simulink model "ATABEY_sistem_modeli"  (R2025b)
settings: Solver=VariableStepAuto  StartTime=0.0  StopTime=simTime  RelTol=1e-3
undefined symbols (not defined in the file or in its folder): uMotorMax, uMotorMin, uServoMax, uServoMin, x0
libraries: aerolibfltsims x1, aerolibanimutils x1
settings Model: Creator=erayacikgz  LastModifiedBy=erayacikgz

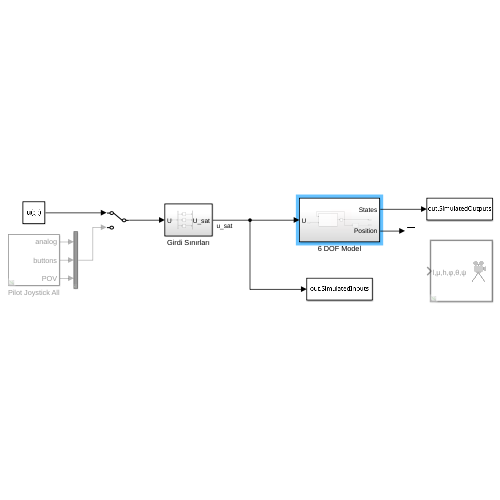
[thumbnail: Simulink's stored preview of the top-level diagram]
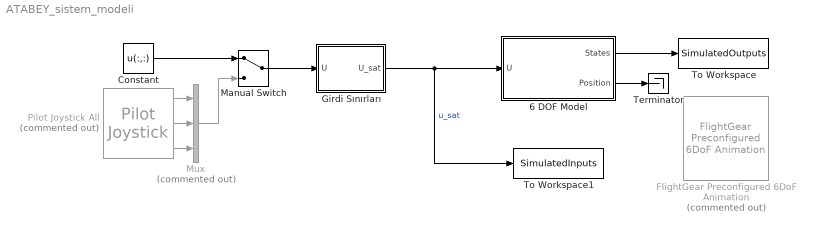
== system ATABEY_sistem_modeli ==
  6 DOF Model : Subsystem
  Constant : Constant  Value=u(:,:)
  FlightGear Preconfigured 6DoF Animation : aerolibfltsims/FlightGear Preconfigured 6DoF Animation  Commented=on  xFlightGearVersion=v2019.1  DestinationIpAddress=127.0.0.1  DestinationPort=5502  SampleTime=1/30  packetVersion=24
  Girdi Sınırları : Subsystem
  Manual Switch : ManualSwitch
  Mux : Mux  Commented=on  Inputs=3
  Pilot Joystick All : aerolibanimutils/Pilot Joystick  Commented=on  JoystickID=Joystick1  OutputConfiguration=AllOutputs  SampleTime=1/30
      settings: LibrarySourceBlock=aerolibanimutils/Pilot Joystick All
  Terminator : Terminator
  To Workspace : ToWorkspace  VariableName=SimulatedOutputs  SaveFormat=Timeseries  SampleTime=-1
  To Workspace1 : ToWorkspace  VariableName=SimulatedInputs  SaveFormat=Timeseries  SampleTime=-1
  wires:
  6 DOF Model/1(States) -> To Workspace/1
  Manual Switch/1 -> Girdi Sınırları/1(U)
  Constant/1 -> Manual Switch/1
  Pilot Joystick All/1 -> Mux/1
  Pilot Joystick All/2 -> Mux/2
  Pilot Joystick All/3 -> Mux/3
  Mux/1 -> Manual Switch/2
  6 DOF Model/2(Position) -> Terminator/1
  Girdi Sınırları/1(U_sat) -> To Workspace1/1, 6 DOF Model/1(U)  "u_sat"

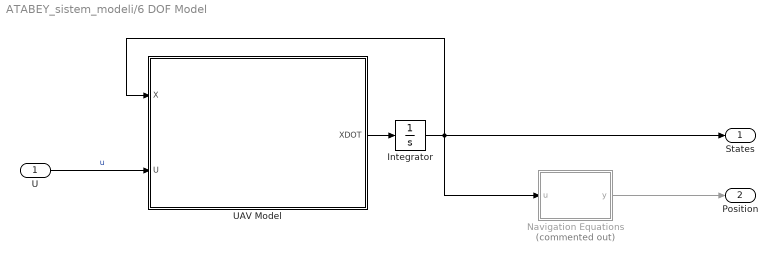
== system ATABEY_sistem_modeli/6 DOF Model ==
  U : Inport
  Integrator : Integrator  InitialCondition=x0(:,:)
  Navigation Equations : MATLAB Function  Commented=on  TreatAsAtomicUnit=on
  UAV Model : MATLAB Function  TreatAsAtomicUnit=on
  States : Outport
  Position : Outport  Port=2
  wires:
  U/1 -> UAV Model/2(U)  "u"
  Navigation Equations/1(y) -> Position/1
  UAV Model/1(XDOT) -> Integrator/1
  Integrator/1 -> States/1, Navigation Equations/1(u), UAV Model/1(X)

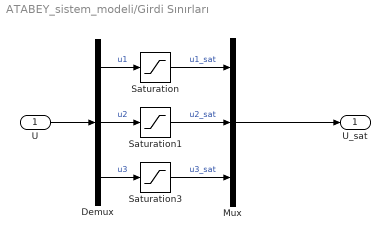
== system ATABEY_sistem_modeli/Girdi Sınırları ==
  U : Inport
  Demux : Demux  Outputs=3
  Mux : Mux  Inputs=3
  Saturation : Saturate  UpperLimit=uServoMax  LowerLimit=uServoMin
  Saturation1 : Saturate  UpperLimit=uServoMax  LowerLimit=uServoMin
  Saturation3 : Saturate  UpperLimit=uMotorMax  LowerLimit=uMotorMin
  U_sat : Outport
  wires:
  Mux/1 -> U_sat/1
  Demux/2 -> Saturation1/1  "u2"
  Saturation/1 -> Mux/1  "u1_sat"
  Saturation3/1 -> Mux/3  "u3_sat"
  U/1 -> Demux/1
  Demux/1 -> Saturation/1  "u1"
  Demux/3 -> Saturation3/1  "u3"
  Saturation1/1 -> Mux/2  "u2_sat"

== matlab function ATABEY_sistem_modeli/6 DOF Model/UAV Model ==
  data: X input double size=[9 1]; XDOT output double size=[9 1]; U input double size=[3 1]
function XDOT = ATABEY_model(X, U)

    XDOT = ATABEY_dynamics(X, U);
    
end

== matlab function ATABEY_sistem_modeli/6 DOF Model/Navigation Equations ==
  data: u input; y output
function y = NAV_eqs(u)

y = u;
